simulink model "MGpa164model"  (R2020a)
settings: Solver=VariableStepAuto  StartTime=0.0  StopTime=0.001  RelTol=1e-3
undefined symbols (not defined in the file): CF, CG, RF, RG
settings Model: DataDictionary=pa164.sldd  Creator=mgesuale  LastModifiedBy=mgesuale

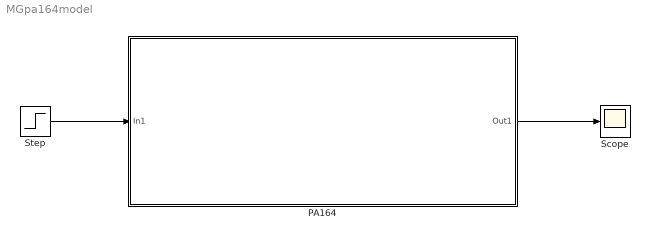
== system MGpa164model ==
  PA164 : Subsystem
  Scope : Scope
  Step : Step  Time=50e-6  After=-.1  SampleTime=4e-9
  wires:
  PA164/1(Out1) -> Scope/1
  Step/1 -> PA164/1(In1)

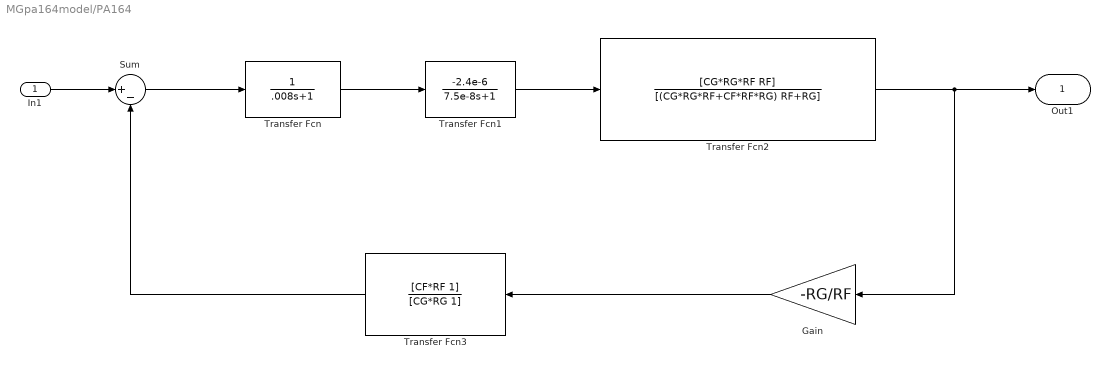
== system MGpa164model/PA164 ==
  In1 : Inport
  Gain : Gain  Gain=-RG/RF
  Sum : Sum  Inputs=|+-
  Transfer Fcn : TransferFcn  Denominator=[.008 1]
  Transfer Fcn1 : TransferFcn  Numerator=[-2.4e-6]  Denominator=[7.5e-8 1]
  Transfer Fcn2 : TransferFcn  Numerator=[CG*RG*RF RF]  Denominator=[(CG*RG*RF+CF*RF*RG) RF+RG]
  Transfer Fcn3 : TransferFcn  Numerator=[CF*RF 1]  Denominator=[CG*RG 1]
  Out1 : Outport
  wires:
  Transfer Fcn2/1 -> Out1/1, Gain/1
  Transfer Fcn3/1 -> Sum/2
  Transfer Fcn1/1 -> Transfer Fcn2/1
  In1/1 -> Sum/1
  Gain/1 -> Transfer Fcn3/1
  Transfer Fcn/1 -> Transfer Fcn1/1
  Sum/1 -> Transfer Fcn/1
